simulink model "ch7example9"  (Simulink 9.2)
settings: Solver=FixedStepDiscrete  StartTime=0.0  StopTime=5  FixedStep=1e-4  RelTol=1e-3  EnableMultiTasking=on
undefined symbols (not defined in the file): rcosine
libraries: commrandsrc2 x1, commsink2 x1, dspobslib x1, commutil2 x1, dspsigops x1
settings Model: Creator=Administrator  LastModifiedBy=Administrator
settings DataIOCC: SignalLoggingName=sigsOut
settings OptimizationCC: LifeSpan=auto
settings DebuggingCC: SaveWithParameterizedLinksMsg=none  SignalResolutionControl=TryResolveAllWithWarning  MultiTaskDSMMsg=warning  MultiTaskCondExecSysMsg=none  FcnCallInpInsideContextMsg=error  StateNameClashWarn=none  SFUnexpectedBacktrackingDiag=error  SFNoUnconditionalDefaultTransitionDiag=error  SFExecutionAtInitializationDiag=warning
settings HardwareCC: TargetUnknown=on
settings SFSimCC: SimUseLocalCustomCode=on
settings RTWCC: RTWUseLocalCustomCode=on
settings CodeAppCC: StateflowObjectComments=off
settings GRTTargetCC: TargetLangStandard=C99 (ISO)  GeneratePreprocessorConditionals=Use local settings
settings ConfigComp: CovExternalEMLEnable=on

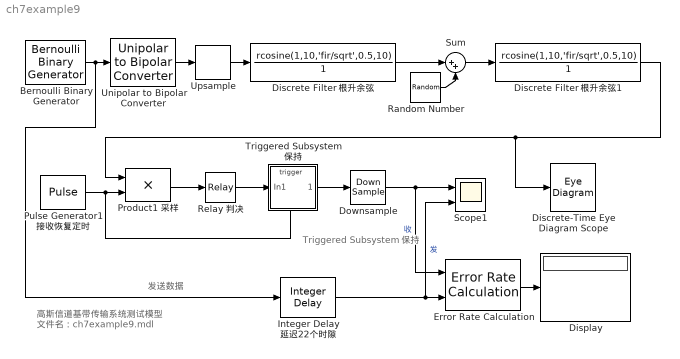
== system ch7example9 ==
  note: 高斯信道基带传输系统测试模型
      | 文件名：ch7example9.mdl
  note: Triggered
      | Subsystem
      | 保持
  note: 发送数据
  Bernoulli Binary Generator : commrandsrc2/Bernoulli Binary Generator  P=0.5  seed=61  Ts=1e-3  frameBased=off  sampPerFrame=1  orient=off  outDataType=double
  Discrete Filter 根升余弦 : DiscreteFilter  Numerator=rcosine(1,10,'fir/sqrt',0.5,10)  Denominator=1  SampleTime=1/10000
  Discrete Filter 根升余弦1 : DiscreteFilter  Numerator=rcosine(1,10,'fir/sqrt',0.5,10)  Denominator=1  SampleTime=1/10000
  Discrete-Time Eye Diagram Scope : EyeDiagram  Tag=EyeDiagram
  Display : Display
  Downsample : DownSample  N=10  InputProcessing=Inherited (this choice will be removed - see release notes)  RateOptions=Allow multirate processing
  Error Rate Calculation : commsink2/Error Rate Calculation  N=0  st_delay=1  cp_mode=Entire frame  subframe=[]  PMode=Port  WsName=ErrorVec  RsMode2=off  stop=off  numErr=100  maxBits=1e6
  Integer Delay 延迟22个时隙 : dspobslib/Integer Delay  delay=22  ic=0  reset_popup=None
      settings: SourceProductName=DSP System Toolbox  SourceProductBaseCode=DS
  Product1 采样 : Product  SaturateOnIntegerOverflow=on  OutDataTypeStr=Inherit: Same as first input
  Pulse Generator1 接收恢复定时 : DiscretePulseGenerator  Period=10  SampleTime=1/10000
  Random Number : RandomNumber  Variance=0.05  SampleTime=0
  Relay 判决 : Relay  OnSwitchValue=0.5  OffSwitchValue=0.5
  Scope1 : Scope  NumInputPorts=2
  Sum : Sum  Inputs=|++  SaturateOnIntegerOverflow=on
  Triggered Subsystem 保持 : Subsystem  TreatAsAtomicUnit=on
  Unipolar to Bipolar Converter : commutil2/Unipolar to Bipolar Converter  M=2  polarity=Positive  dataType=Inherit via internal rule
      settings: SourceProductName=Communications System Toolbox
  Upsample : dspsigops/Upsample  N=10  phase=0  InputProcessing=Columns as channels (frame based)  RateOptions=Allow multirate processing  ic=0  mode=Unused parameter value
  wires:
  Bernoulli Binary Generator/1 -> Unipolar to Bipolar Converter/1, Integer Delay 延迟22个时隙/1
  Unipolar to Bipolar Converter/1 -> Upsample/1
  Upsample/1 -> Discrete Filter 根升余弦/1
  Discrete Filter 根升余弦/1 -> Sum/1
  Random Number/1 -> Sum/2
  Sum/1 -> Discrete Filter 根升余弦1/1
  Pulse Generator1 接收恢复定时/1 -> Product1 采样/2, Triggered Subsystem 保持/Trigger
  Product1 采样/1 -> Relay 判决/1
  Discrete Filter 根升余弦1/1 -> Product1 采样/1, Discrete-Time Eye Diagram Scope/1
  Triggered Subsystem 保持/1(Out1) -> Downsample/1
  Relay 判决/1 -> Triggered Subsystem 保持/1(In1)
  Downsample/1 -> Scope1/1, Error Rate Calculation/1  "收"
  Error Rate Calculation/1 -> Display/1
  Integer Delay 延迟22个时隙/1 -> Error Rate Calculation/2, Scope1/2  "发"

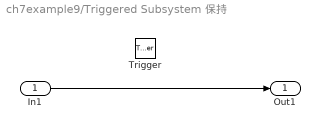
== system ch7example9/Triggered Subsystem 保持 ==
  In1 : Inport
  Trigger : TriggerPort  VariantControl=(inherit)
  Out1 : Outport
  wires:
  In1/1 -> Out1/1
